simulink model "simulation_model"  (R2022b)
settings: Solver=VariableStepAuto  StartTime=0.0  StopTime=1230000  RelTol=1e-3
model workspace (MAT data in the model file):
  cl1 = 125
  cl2 = 40
  cl3 = 30
  dcmax = [2.05 6.15]
  dcmax2 = [2.04 4]
  iba = 10
undefined symbols (not defined in the file or in its folder): Batt, BatteryCback, BatteryLoadFcn, Continuous, DiscIntNeverNeededParam, gcbh, sps_rtmsupport, spsBatteryModel, Ts
libraries: simulink x7, simulink_extras x2, spsControlledVoltageSourceLib x1, spsCurrentMeasurementLib x1, spsSeriesRLCBranchLib x1, spsControlledCurrentSourceLib x1, spspowerguiLib x1
settings Model: Creator=DSPR_Lab1  LastModifiedBy=DSPR_Lab1

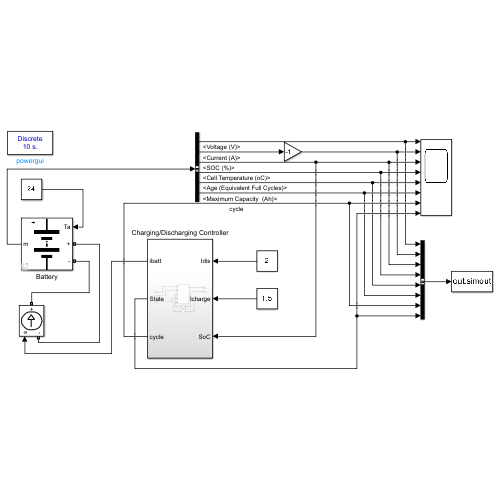
[thumbnail: Simulink's stored preview of the top-level diagram]
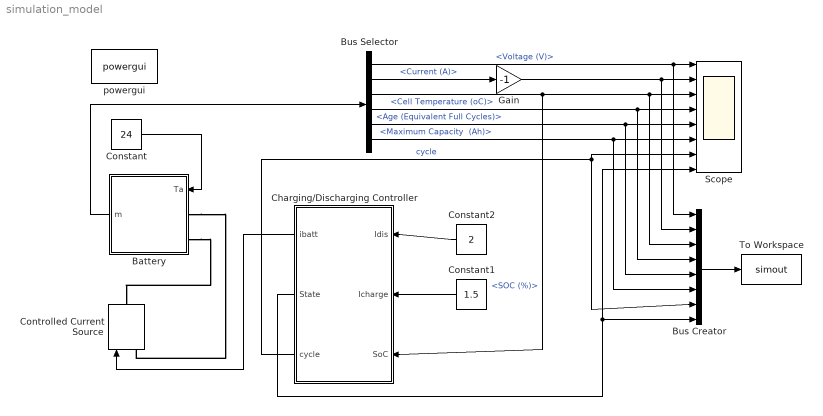
== system simulation_model ==
  Battery : Subsystem  AncestorBlock=sps_lib/Sources/Battery  DialogController=POWERSYS.PowerSysDialog  LoadFcn=sps_rtmsupport('LoadFcn',gcbh); BatteryLoadFcn(gcb)  InitFcn=BatteryCback(gcb,1)  StartFcn=sps_rtmsupport('StartFcn',gcbh);  StopFcn=sps_rtmsupport('StopFcn',gcbh);  mask(Battery){BatType=Lithium-Ion, ShowTempParam=on, ThermalPreset=no, ShowAgeParam=on, NomV=3.3, NomQ=2.05, SOC=0, Batt_Tr=30, PresetModel=off, MaxQ=2.05, MinV=2.75, FullV=4.2, Dis_rate=2, R=.02, Normal_OP=1.9, expZone=[3.38 1.7], current=[.5125 1.025 2.05 4.1 8.2], Units=Ampere-hour, Tci=24, NomT=20, T2=0, MaxQ2=1.85, FullV2=4.1, Normal_OP2=3.3, expZone2=[3.45  1.1], Rca=3, ti=1000, Dp=0, Neq0=iba, Tsim=90, Ta1=20, Qeol=1.49, Reol=0.02*3.2, Char_age=[1.44, 2], Dis_age=[2  6.15], N1=cl1, N2=1600, N3=50, N4=cl2, Ta2=45, N5=cl3}
      mask prompts: BatType "Type:"; ShowTempParam "Simulate temperature effects"; ThermalPreset "Use a preset battery:"; ShowAgeParam "Simulate aging effects"; NomV "Nominal voltage (V)"; NomQ "Rated capacity (Ah)"; SOC "Initial state-of-charge (%)"; Batt_Tr "Battery response time (s)"; PresetModel "Determined from the nominal parameters of the battery"; MaxQ "Maximum capacity (Ah)"; MinV "Cut-off Voltage (V)"; FullV "Fully charged voltage (V)"; Dis_rate "Nominal discharge current (A)"; R "Internal resistance (Ohms)"; Normal_OP "Capacity (Ah) at nominal voltage"; expZone "Exponential zone [Voltage (V), Capacity (Ah)]"; current "Discharge current [i1, i2, i3,...] (A)"; Tci "Initial cell temperature (deg. C)"; NomT "Nominal ambient temperature T1 (deg. C)"; T2 "Second ambient temperature T2 (deg. C)"; MaxQ2 "Maximum capacity (Ah)"; FullV2 "Initial discharge voltage (V)"; Normal_OP2 "Voltage at 90% maximum capacity (V)"; expZone2 "Exponential zone [Voltage (V), Capacity (Ah)]"; Rca "Thermal resistance, cell-to-ambient (deg. C/W)"; ti "Thermal time constant, cell-to-ambient (s)"; Dp "Heat loss difference [charge vs. discharge] (W)"; Neq0 "Initial battery age (Equivalent full cycles)"; Tsim "Aging model sampling time (s)"; Ta1 "Ambient temperature Ta1 (deg. C)"; Qeol "Capacity at EOL (End Of Life) (Ah)"; Reol "Internal resistance at EOL (Ohms)"; Char_age "Charge current (nominal, maximum) [Ic (A), Icmax (A)]"; Dis_age "Discharge current (nominal, maximum) [Id (A), Idmax (A)]"; N1 "Cycle life at 100 % DOD, Ic and Id (Cycles)"; N2 "Cycle life at 25 % DOD, Ic and Id (Cycles)"; N3 "Cycle life at 100 % DOD, Ic and Idmax (Cycles)"; N4 "Cycle life at 100 % DOD, Icmax and Id (Cycles)"; Ta2 "Ambient temperature Ta2 (deg. C)"; N5 "Cycle life at 100 % DOD, Ic and Id (Cycles)"
      mask help: Implements a generic battery model for most popular battery types. Temperature and aging (due to cycling) effects can be specified for Lithium-Ion battery type.
      mask init:
      | block = gcb;
      | BatteryCback(block,3)
      | [Batt BT, WantBlockChoice, Ts] = BatteryParam(NomV,NomQ,MaxQ,MinV,FullV,Dis_rate,R,Normal_OP,expZone,block,0);
      | powericon('SetInternalModels','set',block,WantBlockChoice);
      | BatteryCback(block,1);
      settings: LibrarySourceBlock=sps_lib/Sources/Battery  CopyFcn=sps_rtmsupport('CopyFcn',gcbh);  DeleteFcn=sps_rtmsupport('DeleteFcn',gcbh);  UndoDeleteFcn=sps_rtmsupport('UndoDeleteFcn',gcbh);  ModelCloseFcn=sps_rtmsupport('ModelCloseFcn',gcbh);  PreSaveFcn=sps_rtmsupport('PreSaveFcn',gcbh);  PostSaveFcn=sps_rtmsupport('PostSaveFcn',gcbh);  NameChangeFcn=sps_rtmsupport('NameChangeFcn',gcbh);  PreCopyFcn=sps_rtmsupport('PreCopyFcn',gcbh);  OpenFcn=sps_rtmsupport('OpenFcn',gcbh, [1,2,3,4,9,18]);  CloseFcn=sps_rtmsupport('CloseFcn',gcbh);  PreDeleteFcn=sps_rtmsupport('PreDeleteFcn',gcbh);
      mask Help: helpview(psbhelp)
      mask TypeOptions BatType: Lead-Acid | Lithium-Ion | Nickel-Cadmium | Nickel-Metal-Hydride
      mask Callback BatType: BatteryCback(gcb,1)
      mask Callback ShowTempParam: BatteryCback(gcb,1)
      mask TypeOptions ThermalPreset: no | 3.3V  2.3Ah  (LiFePO4) | 3.6V  2050mAh   (LiCoO2) | 3.6V  2.0Ah | 3.6V  3.6Ah  (LiNiO2) | 3.6V  4.5Ah | 3.6V  48Ah  (LiNiO2) | 3.7V  4.4Ah | 7.4V  5.4Ah  (LiCoO2) | 11.1V  6600mAh  (LiCoO2) | 12.8V  40Ah  (LiFeMgPO4)
      mask Callback ThermalPreset: BatteryCback(gcb,4)
      mask Callback ShowAgeParam: BatteryCback(gcb,1)
      mask Callback PresetModel: BatteryCback(gcb,1)
      mask TypeOptions Units: Ampere-hour | Time
      mask Callback ti: sps_rtmsupport('parametereditingmodes',gcbh, [1,2,3,4,9,18]);
      mask DialogControl ParameterTabVar0 Prompt: Parameters
      mask DialogControl Tempcontainer Prompt: Temperature
      mask DialogControl Agecontainer Prompt: Aging
      mask DialogControl ParameterTabVar01 Prompt: Discharge
      mask DialogControl Container9 Prompt: Display characteristics
      mask DialogControl PlotButton Prompt: Plot
      mask DialogControl PlotButton Callback: BatteryCback(gcb,0)
      mask DialogControl Temperature Prompt: Temperature
      mask DialogControl Container7 Prompt: Discharge parameters at T2
      mask DialogControl Container8 Prompt: Thermal response and Heat loss
      mask DialogControl Aging Prompt: Aging
      mask DialogControl Container16 Prompt: Aging characteristics at ambient temperature Ta1
      mask DialogControl Container13 Prompt: Aging characteristics at ambient temperature Ta2
  Bus Creator : BusCreator  Inputs=8
  Bus Selector : BusSelector  OutputSignals="Voltage (V),Current (A),SOC (%),Cell Temperature (oC),Age (Equivalent Full Cycles),Maximum Capacity  (Ah)"
  Charging/Discharging Controller : Subsystem
  Constant : Constant  Value=24
  Constant1 : Constant  Value=1.5
  Constant2 : Constant  Value=2
  Controlled Current Source : spsControlledCurrentSourceLib/Controlled Current Source  Initialize=on  Source_Type=AC  Amplitude=0  Phase=0  Frequency=0  Measurements=None
  Gain : Gain  Gain=-1
  Scope : Scope  NumInputPorts=8
  To Workspace : ToWorkspace  VariableName=simout  SampleTime=-1
  powergui : spspowerguiLib/powergui  Priority=1  SimulationMode=Discrete  SampleTime=10  frequency=60  Iterations=50  frequencyindice=0  Pbase=100e6  ErrMax=1e-4  UnitsV=kV  UnitsW=MW  buscounter=0  FunctionMessages=off  echomessages=off  EnableUseOfTLC=off  CurrentSourceSwitches=on  DisableSnubberDevices=off  DisableRonSwitches=off  DisableVfSwitches=off  DisplayEquations=off  AutomaticDiscreteSolvers=off  SolverType=Tustin/Backward Euler (TBE)  Interpol=off  ExternalGateDelay=off  methode=off  Ts=100  x0status=blocks  SPID=on  SwTol=0  HookPort=off  NonlinearTolerance=1e-4  nMaxIteration=100  ContinueOnMaxIteration=off  RestoreLinks=warning  ResistiveCurrentMeasurement=off  Frange=[0:2:500]  Ylog=off  Xlog=on  ShowGrid=off  save=off  variable=ZData  structure=0  ZoomFFT=off  StartTime=0.0  cycles=1  DisplayStyle=1  fundamental=60  FreqAxis=off  MaxFrequency=1000  frequencyindicesteady=1  RmsSteady=1  display=off
  wires:
  Charging/Discharging Controller/3(cycle) -> Bus Creator/7, Scope/7  "cycle"
  Bus Selector/2 -> Gain/1  "<Current (A)>"
  Charging/Discharging Controller/2(State) -> Scope/8, Bus Creator/8
  Constant1/1 -> Charging/Discharging Controller/2(Icharge)
  Constant/1 -> Battery/1(Ta)
  Charging/Discharging Controller/1(ibatt) -> Controlled Current Source/1
  Constant2/1 -> Charging/Discharging Controller/1(Idis)
  Bus Creator/1 -> To Workspace/1
  Battery/1(m) -> Bus Selector/1
  Bus Selector/1 -> Bus Creator/1, Scope/1  "<Voltage (V)>"
  Gain/1 -> Bus Creator/2, Scope/2
  Bus Selector/3 -> Charging/Discharging Controller/3(SoC), Bus Creator/3, Scope/3  "<SOC (%)>"
  Bus Selector/4 -> Bus Creator/4, Scope/4  "<Cell Temperature (oC)>"
  Bus Selector/5 -> Bus Creator/5, Scope/5  "<Age (Equivalent Full Cycles)>"
  Bus Selector/6 -> Bus Creator/6, Scope/6  "<Maximum Capacity  (Ah)>"
  connections:
  Battery/LConn2 -- Controlled Current Source/RConn1
  Battery/LConn1 -- Controlled Current Source/LConn1

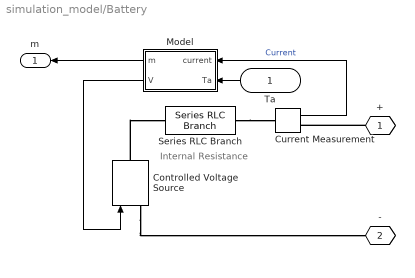
== system simulation_model/Battery ==
  note: Internal Resistance
  Ta : Inport
  Controlled Voltage Source : spsControlledVoltageSourceLib/Controlled Voltage Source  Initialize=on  Source_Type=AC  Amplitude=0  Phase=0  Frequency=0  Measurements=None
  Current Measurement : spsCurrentMeasurementLib/Current Measurement  PhasorSimulation=off  OutputType=Complex  PSBequivalent=0
  Model : Subsystem  AncestorBlock=spsBatteryModel/Continuous
      settings: LibrarySourceBlock=spsBatteryModel/Continuous
  Series RLC Branch : spsSeriesRLCBranchLib/Series RLC Branch  LConnTagsString=__new0  RConnTagsString=__new0  BranchType=R  Resistance=Batt.R  Inductance=1e-3  SetiL0=off  InitialCurrent=0  Capacitance=1e-6  Setx0=off  InitialVoltage=0  Measurements=None
  + : PMIOPort  Tag=PMCPort  Side=Left
  - : PMIOPort  Tag=PMCPort  Port=2  Side=Left
  m : Outport  VectorParamsAs1DForOutWhenUnconnected=off
  wires:
  Model/2(V) -> Controlled Voltage Source/1
  Model/1(m) -> m/1
  Current Measurement/1 -> Model/1(current)  "Current"
  Ta/1 -> Model/2(Ta)
  connections:
  +/RConn1 -- Current Measurement/RConn1
  Controlled Voltage Source/LConn1 -- -/RConn1
  Controlled Voltage Source/RConn1 -- Series RLC Branch/LConn1
  Series RLC Branch/RConn1 -- Current Measurement/LConn1

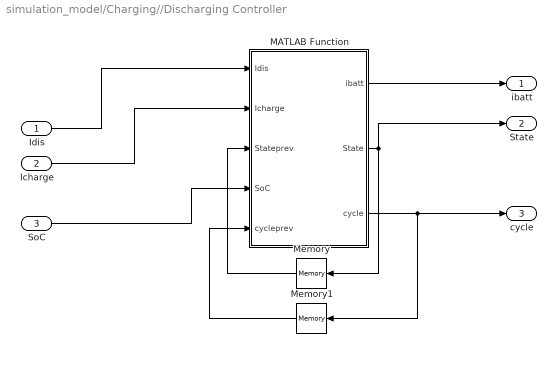
== system simulation_model/Charging//Discharging Controller ==
  Idis : Inport
  Icharge : Inport  Port=2
  SoC : Inport  Port=3
  MATLAB Function : MATLAB Function  TreatAsAtomicUnit=on
  Memory : Memory
  Memory1 : Memory
  ibatt : Outport
  State : Outport  Port=2
  cycle : Outport  Port=3
  wires:
  Idis/1 -> MATLAB Function/1(Idis)
  Icharge/1 -> MATLAB Function/2(Icharge)
  Memory/1 -> MATLAB Function/3(Stateprev)
  MATLAB Function/2(State) -> Memory/1, State/1
  MATLAB Function/1(ibatt) -> ibatt/1
  SoC/1 -> MATLAB Function/4(SoC)
  MATLAB Function/3(cycle) -> cycle/1, Memory1/1
  Memory1/1 -> MATLAB Function/5(cycleprev)

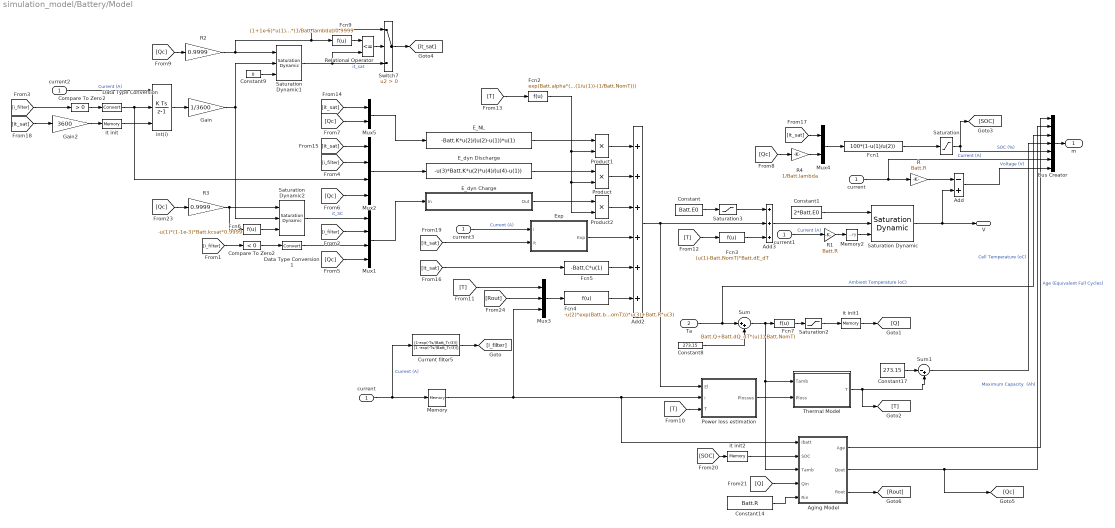
== system simulation_model/Battery/Model ==
  current : Inport
  Ta : Inport  Port=2
  Add : Sum  Inputs=-+
  Add2 : Sum  Inputs=++++++
  Add3 : Sum  Inputs=+++
  Aging Model : Subsystem  AncestorBlock=spsBatteryModel/Aging Model
      settings: LibrarySourceBlock=spsBatteryModel/Aging Model
  Bus Creator : BusCreator  Inputs=7
  Compare To Zero : simulink/Logic and Bit Operations/Compare To Zero  relop=>  OutDataTypeStr=uint8
  Compare To Zero2 : simulink/Logic and Bit Operations/Compare To Zero  relop=<  OutDataTypeStr=uint8
  Constant : Constant  Value=Batt.E0
  Constant1 : Constant  Value=2*Batt.E0
  Constant14 : Constant  Value=Batt.R
  Constant17 : Constant  Value=273.15
  Constant8 : Constant  Value=273.15
  Constant9 : Constant  Value=0
  Current filter5 : DiscreteTransferFcn  Numerator=[1-exp(-Ts/(Batt_Tr/3))]  Denominator=[1 -exp(-Ts/(Batt_Tr/3))]  SampleTime=Ts
  Data Type Conversion1 : DataTypeConversion  SaturateOnIntegerOverflow=off  RndMeth=Floor
  Data Type Conversion2 : DataTypeConversion  SaturateOnIntegerOverflow=off  RndMeth=Floor
  E_NL : Fcn  Expr=-Batt.K*u(2)/(u(2)-u(1))*u(1)
  E_dyn Charge : Subsystem
  E_dyn Discharge : Fcn  Expr=-u(3)*Batt.K*u(2)*u(4)/(u(4)-u(1))
  Exp : Subsystem
  Fcn1 : Fcn  Expr=100*(1-u(1)/u(2))
  Fcn2 : Fcn  Expr=exp(Batt.alpha*((1/u(1))-(1/Batt.NomT)))
  Fcn3 : Fcn  Expr=(u(1)-Batt.NomT)*Batt.dE_dT
  Fcn4 : Fcn  Expr=-u(2)*exp(Batt.beta*((1/u(1))-(1/Batt.NomT)))*u(3)+Batt.R*u(3)
  Fcn5 : Fcn  Expr=-Batt.C*u(1)
  Fcn6 : Fcn  Expr=-u(1)*(1-1e-3)*Batt.kcsat*0.9999
  Fcn7 : Fcn  Expr=Batt.Q+Batt.dQ_dT*(u(1)-Batt.NomT)
  Fcn9 : Fcn  Expr=(1+1e-6)*u(1)*(1/Batt.lambda)/0.9999
  Gain : Gain  Gain=1/3600
  Gain2 : Gain  Gain=3600
  Memory : Memory
  Memory2 : Memory  InheritSampleTime=on
  Mux1 : Mux
  Mux2 : Mux
  Mux3 : Mux  Inputs=3
  Mux4 : Mux  Inputs=2
  Mux5 : Mux  Inputs=2
  Power loss estimation : Subsystem
  Product : Product
  Product1 : Product
  Product2 : Product
  R : Gain  Gain=Batt.R
  R1 : Gain  Gain=Batt.R
  R2 : Gain  Gain=0.9999
  R3 : Gain  Gain=0.9999
  R4 : Gain  Gain=1/Batt.lambda
  Relational Operator : RelationalOperator  Operator=<=  RndMeth=Simplest  InputSameDT=off
  Saturation : Saturate  UpperLimit=100  LowerLimit=0
  Saturation Dynamic : simulink/Discontinuities/Saturation Dynamic  OutMin=[]  OutMax=[]  OutDataTypeStr=Inherit: Same as second input  OutDataType=sfix(16)  OutScaling=2^-10  DoSatur=off
  Saturation Dynamic1 : simulink/Discontinuities/Saturation Dynamic  OutMin=[]  OutMax=[]  OutDataTypeStr=Inherit: Same as second input  OutDataType=sfix(16)  OutScaling=2^-10  DoSatur=off
  Saturation Dynamic2 : simulink/Discontinuities/Saturation Dynamic  OutMin=[]  OutMax=[]  OutDataTypeStr=Inherit: Same as second input  OutDataType=sfix(16)  OutScaling=2^-10  DoSatur=off
  Saturation2 : Saturate  UpperLimit=max(NomQ,MaxQ)  LowerLimit=0
  Saturation3 : Saturate  UpperLimit=Batt.Va-Batt.dE_dT*(Batt.Tci-Batt.NomT)-Batt.A  LowerLimit=-inf
  Sum : Sum  Inputs=|++
  Sum1 : Sum  Inputs=|-+
  Switch7 : Switch  Criteria=u2 > Threshold  SaturateOnIntegerOverflow=off  InputSameDT=off
  Thermal Model : Subsystem  VariantControl=Discrete
  "current " : InportShadow
  current1 : InportShadow
  current2 : InportShadow
  current3 : InportShadow
  int(i) : DiscreteIntegrator  ExternalReset=rising  InitialConditionSource=external  SampleTime=Ts  LimitOutput=on  UpperSaturationLimit=Batt.Qmax*3600  ICPrevOutput=DiscIntNeverNeededParam  ICPrevScaledInput=DiscIntNeverNeededParam
  it init : Memory  InitialCondition=(1-SOC/100)*Batt.Q*(1/Batt.lambda)*3600
  it init1 : Memory  InitialCondition=MaxQ
  it init2 : Memory  InitialCondition=SOC
  m : Outport  VectorParamsAs1DForOutWhenUnconnected=off
  V : Outport  Port=2  VectorParamsAs1DForOutWhenUnconnected=off
  wires:
  current/1 -> Bus Creator/6, R/1  "Current (A)"
  int(i)/1 -> Gain/1
  Fcn1/1 -> Saturation/1
  Add/1 -> Bus Creator/7  "Voltage (V)"
  R/1 -> Add/1
  Bus Creator/1 -> m/1
  Mux2/1 -> E_dyn Discharge/1
  Constant/1 -> Saturation3/1
  Mux1/1 -> E_dyn Charge/1(In)
  it init/1 -> int(i)/3
  Compare To Zero/1 -> Data Type Conversion2/1
  Compare To Zero2/1 -> Data Type Conversion1/1
  Data Type Conversion2/1 -> Mux2/3, int(i)/2
  Gain2/1 -> it init/1
  Exp/1(Exp) -> Add2/4
  Data Type Conversion1/1 -> Mux1/3
  Saturation Dynamic2/1 -> Mux1/1  "it_SC"
  Constant1/1 -> Saturation Dynamic/1
  Add3/1 -> Saturation Dynamic/2
  E_dyn Discharge/1 -> Product/1
  Product/1 -> Add2/2
  E_NL/1 -> Product1/1
  Product1/1 -> Add2/1
  Memory/1 -> Mux3/3, Aging Model/1(Ibatt), Power loss estimation/2(i)
  Power loss estimation/1(Plosses) -> Thermal Model/2(Ploss)
  Fcn2/1 -> Product2/2, Product/2, Product1/2
  Fcn4/1 -> Add2/6
  Mux3/1 -> Fcn4/1
  E_dyn Charge/1(Out) -> Product2/1
  Product2/1 -> Add2/3
  Fcn5/1 -> Add2/5
  Ta/1 -> Sum/1, Bus Creator/3  "Ambient Temperature (oC)"
  Constant8/1 -> Sum/2
  Mux4/1 -> Fcn1/1
  Mux5/1 -> E_NL/1
  Fcn3/1 -> Add3/3
  Fcn6/1 -> Saturation Dynamic2/3
  Sum/1 -> Aging Model/3(Tamb), Thermal Model/1(Tamb), Fcn7/1
  Fcn7/1 -> Saturation2/1
  Saturation3/1 -> Add3/1
  Saturation2/1 -> it init1/1
  current2/1 -> int(i)/1  "Current (A)"
  current3/1 -> Exp/1(i)  "Current (A)"
  "current "/1 -> Current filter5/1, Memory/1  "Current (A)"
  Current filter5/1 -> [i_filter]
  [i_filter] -> Compare To Zero2/1
  [i_filter] -> Mux1/2
  [i_filter] -> Compare To Zero/1
  [i_filter] -> Mux2/2
  it init1/1 -> [Q]
  [Qc] -> Mux1/4
  [Qc] -> Mux2/4
  [Qc] -> R4/1
  [Qc] -> R2/1
  [T] -> Mux3/1
  [T] -> Fcn3/1
  [T] -> Fcn2/1
  [it_sat] -> Mux5/1
  [it_sat] -> Mux2/1
  [it_sat] -> Fcn5/1
  [it_sat] -> Mux4/1
  [it_sat] -> Gain2/1
  [it_sat] -> Exp/2(it)
  [Qc] -> R3/1
  R3/1 -> Fcn6/1, Saturation Dynamic2/1
  Add2/1 -> Power loss estimation/1(El), Add3/2
  [T] -> Power loss estimation/3(T)
  R4/1 -> Mux4/2
  Saturation/1 -> Bus Creator/5, [SOC]  "SOC (%)"
  Saturation Dynamic/1 -> V/1, Add/2
  [Qc] -> Mux5/2
  [SOC] -> it init2/1
  [Q] -> Aging Model/4(Qin)
  Aging Model/2(Qout) -> Bus Creator/2, [Qc]  "Maximum Capacity  (Ah)"
  Constant14/1 -> Aging Model/5(Rin)
  Aging Model/3(Rout) -> [Rout]
  [Rout] -> Mux3/2
  Aging Model/1(Age) -> Bus Creator/1  "Age (Equivalent Full Cycles)"
  it init2/1 -> Aging Model/2(SOC)
  Gain/1 -> Saturation Dynamic1/2, Saturation Dynamic2/2
  Constant9/1 -> Saturation Dynamic1/3
  current1/1 -> R1/1  "Current (A)"
  Memory2/1 -> Saturation Dynamic/3
  R1/1 -> Memory2/1
  Saturation Dynamic1/1 -> Relational Operator/2, Switch7/3  "it_sat"
  R2/1 -> Switch7/1, Fcn9/1, Saturation Dynamic1/1
  Switch7/1 -> [it_sat]
  Fcn9/1 -> Relational Operator/1
  Relational Operator/1 -> Switch7/2
  Constant17/1 -> Sum1/1
  Thermal Model/1(T) -> Sum1/2, [T]
  Sum1/1 -> Bus Creator/4  "Cell Temperature (oC)"

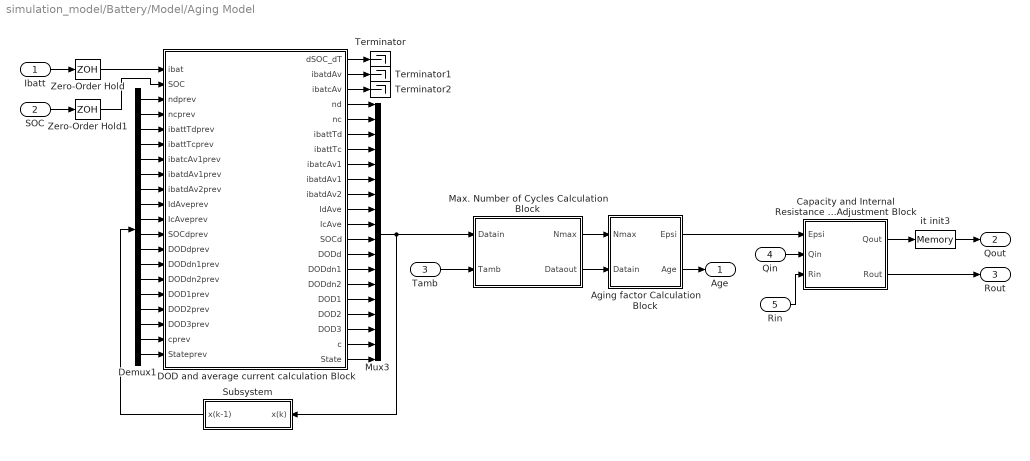
== system simulation_model/Battery/Model/Aging Model ==
  Ibatt : Inport
  SOC : Inport  Port=2
  Tamb : Inport  Port=3
  Qin : Inport  Port=4
  Rin : Inport  Port=5
  Aging factor Calculation Block : Subsystem
  Capacity and Internal Resistance Adjustment Block : Subsystem
  DOD and average current calculation Block : MATLAB Function  TreatAsAtomicUnit=on
  Demux1 : Demux  Outputs=18
      settings: DisplayOption=none
  Max. Number of Cycles Calculation Block : Subsystem
  Mux3 : Mux  Inputs=18
  Subsystem : Subsystem
  Terminator : Terminator
  Terminator1 : Terminator
  Terminator2 : Terminator
  Zero-Order Hold : ZeroOrderHold  SampleTime=Batt.Tsim
  Zero-Order Hold1 : ZeroOrderHold  SampleTime=Batt.Tsim
  it init3 : Memory  InitialCondition=MaxQ
  Age : Outport  VectorParamsAs1DForOutWhenUnconnected=off
  Qout : Outport  Port=2  VectorParamsAs1DForOutWhenUnconnected=off
  Rout : Outport  Port=3  VectorParamsAs1DForOutWhenUnconnected=off
  wires:
  it init3/1 -> Qout/1
  Zero-Order Hold1/1 -> DOD and average current calculation Block/2(SOC)
  Zero-Order Hold/1 -> DOD and average current calculation Block/1(ibat)
  Aging factor Calculation Block/2(Age) -> Age/1
  SOC/1 -> Zero-Order Hold1/1
  Ibatt/1 -> Zero-Order Hold/1
  Max. Number of Cycles Calculation Block/2(Dataout) -> Aging factor Calculation Block/2(Datain)
  Max. Number of Cycles Calculation Block/1(Nmax) -> Aging factor Calculation Block/1(Nmax)
  Demux1/5 -> DOD and average current calculation Block/7(ibatcAv1prev)
  DOD and average current calculation Block/2(ibatdAv) -> Terminator1/1
  DOD and average current calculation Block/3(ibatcAv) -> Terminator2/1
  DOD and average current calculation Block/1(dSOC_dT) -> Terminator/1
  Demux1/2 -> DOD and average current calculation Block/4(ncprev)
  Subsystem/1(x(k-1)) -> Demux1/1
  Demux1/1 -> DOD and average current calculation Block/3(ndprev)
  DOD and average current calculation Block/18(DOD2) -> Mux3/15
  DOD and average current calculation Block/12(IcAve) -> Mux3/9
  DOD and average current calculation Block/17(DOD1) -> Mux3/14
  Demux1/8 -> DOD and average current calculation Block/10(IdAveprev)
  Demux1/14 -> DOD and average current calculation Block/16(DOD1prev)
  DOD and average current calculation Block/8(ibatcAv1) -> Mux3/5
  Demux1/4 -> DOD and average current calculation Block/6(ibattTcprev)
  DOD and average current calculation Block/7(ibattTc) -> Mux3/4
  DOD and average current calculation Block/11(IdAve) -> Mux3/8
  DOD and average current calculation Block/19(DOD3) -> Mux3/16
  DOD and average current calculation Block/10(ibatdAv2) -> Mux3/7
  DOD and average current calculation Block/14(DODd) -> Mux3/11
  Demux1/7 -> DOD and average current calculation Block/9(ibatdAv2prev)
  Demux1/15 -> DOD and average current calculation Block/17(DOD2prev)
  DOD and average current calculation Block/6(ibattTd) -> Mux3/3
  Demux1/11 -> DOD and average current calculation Block/13(DODdprev)
  DOD and average current calculation Block/20(c) -> Mux3/17
  Demux1/18 -> DOD and average current calculation Block/20(Stateprev)
  DOD and average current calculation Block/13(SOCd) -> Mux3/10
  DOD and average current calculation Block/21(State) -> Mux3/18
  DOD and average current calculation Block/15(DODdn1) -> Mux3/12
  DOD and average current calculation Block/5(nc) -> Mux3/2
  Demux1/17 -> DOD and average current calculation Block/19(cprev)
  Demux1/16 -> DOD and average current calculation Block/18(DOD3prev)
  Demux1/9 -> DOD and average current calculation Block/11(IcAveprev)
  Demux1/12 -> DOD and average current calculation Block/14(DODdn1prev)
  Demux1/6 -> DOD and average current calculation Block/8(ibatdAv1prev)
  DOD and average current calculation Block/16(DODdn2) -> Mux3/13
  DOD and average current calculation Block/4(nd) -> Mux3/1
  Demux1/13 -> DOD and average current calculation Block/15(DODdn2prev)
  Demux1/3 -> DOD and average current calculation Block/5(ibattTdprev)
  Demux1/10 -> DOD and average current calculation Block/12(SOCdprev)
  DOD and average current calculation Block/9(ibatdAv1) -> Mux3/6
  Tamb/1 -> Max. Number of Cycles Calculation Block/2(Tamb)
  Capacity and Internal Resistance Adjustment Block/1(Qout) -> it init3/1
  Qin/1 -> Capacity and Internal Resistance Adjustment Block/2(Qin)
  Rin/1 -> Capacity and Internal Resistance Adjustment Block/3(Rin)
  Capacity and Internal Resistance Adjustment Block/2(Rout) -> Rout/1
  Aging factor Calculation Block/1(Epsi) -> Capacity and Internal Resistance Adjustment Block/1(Epsi)
  Mux3/1 -> Max. Number of Cycles Calculation Block/1(Datain), Subsystem/1(x(k))

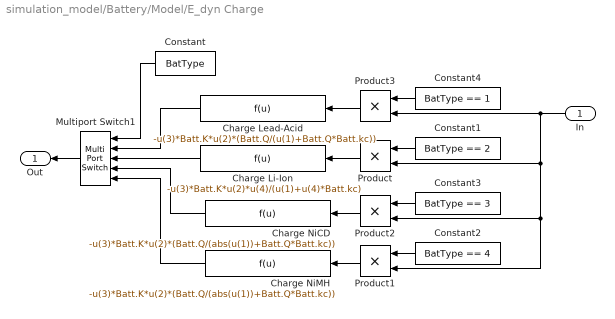
== system simulation_model/Battery/Model/E_dyn Charge ==
  In : Inport
  Charge Lead-Acid : Fcn  Expr=-u(3)*Batt.K*u(2)*(Batt.Q/(u(1)+Batt.Q*Batt.kc))
  Charge Li-Ion : Fcn  Expr=-u(3)*Batt.K*u(2)*u(4)/(u(1)+u(4)*Batt.kc)
  Charge NiCD : Fcn  Expr=-u(3)*Batt.K*u(2)*(Batt.Q/(abs(u(1))+Batt.Q*Batt.kc))
  Charge NiMH : Fcn  Expr=-u(3)*Batt.K*u(2)*(Batt.Q/(abs(u(1))+Batt.Q*Batt.kc))
  Constant : Constant  Value=BatType
  Constant1 : Constant  Value=BatType == 2  OutDataTypeStr=double
  Constant2 : Constant  Value=BatType == 4  OutDataTypeStr=double
  Constant3 : Constant  Value=BatType == 3  OutDataTypeStr=double
  Constant4 : Constant  Value=BatType == 1  OutDataTypeStr=double
  Multiport Switch1 : MultiPortSwitch  Inputs=4  SaturateOnIntegerOverflow=off  InputSameDT=off
  Product{,1..3} (4 alike) : Product  RndMeth=Zero
  Out : Outport  VectorParamsAs1DForOutWhenUnconnected=off
  wires:
  Multiport Switch1/1 -> Out/1
  Charge Li-Ion/1 -> Multiport Switch1/3
  Charge NiMH/1 -> Multiport Switch1/5
  Charge NiCD/1 -> Multiport Switch1/4
  Charge Lead-Acid/1 -> Multiport Switch1/2
  Constant/1 -> Multiport Switch1/1
  In/1 -> Product3/2, Product/2, Product1/2, Product2/2
  Product/1 -> Charge Li-Ion/1
  Constant1/1 -> Product/1
  Product1/1 -> Charge NiMH/1
  Constant2/1 -> Product1/1
  Product2/1 -> Charge NiCD/1
  Constant3/1 -> Product2/1
  Product3/1 -> Charge Lead-Acid/1
  Constant4/1 -> Product3/1

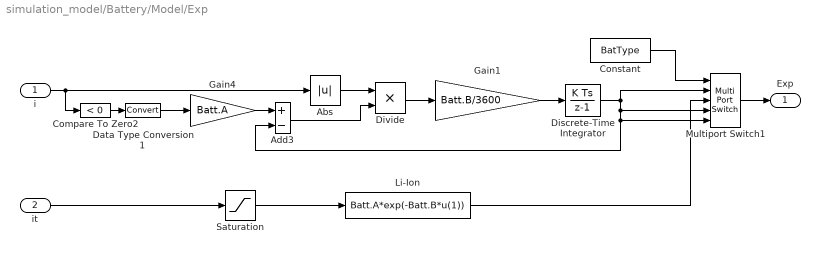
== system simulation_model/Battery/Model/Exp ==
  i : Inport
  it : Inport  Port=2
  Abs : Abs  SaturateOnIntegerOverflow=off
  Add3 : Sum  Inputs=+-
  Compare To Zero2 : simulink/Logic and Bit Operations/Compare To Zero  relop=<  OutDataTypeStr=uint8
  Constant : Constant  Value=BatType
  Data Type Conversion1 : DataTypeConversion  SaturateOnIntegerOverflow=off  RndMeth=Floor
  Discrete-Time Integrator : DiscreteIntegrator  InitialCondition=Batt.A*exp(-Batt.B*(1-SOC/100)*Batt.Q)  SampleTime=Ts  ICPrevOutput=DiscIntNeverNeededParam  ICPrevScaledInput=DiscIntNeverNeededParam
  Divide : Product  Inputs=**
  Gain1 : Gain  Gain=Batt.B/3600
  Gain4 : Gain  Gain=Batt.A
  Li-Ion : Fcn  Expr=Batt.A*exp(-Batt.B*u(1))
  Multiport Switch1 : MultiPortSwitch  Inputs=4  SaturateOnIntegerOverflow=off  InputSameDT=off
  Saturation : Saturate  UpperLimit=Batt.Qmax*(1/Batt.lambda)  LowerLimit=-inf
  Exp : Outport  VectorParamsAs1DForOutWhenUnconnected=off
  wires:
  Discrete-Time Integrator/1 -> Multiport Switch1/2, Multiport Switch1/4, Add3/2, Multiport Switch1/5
  Gain4/1 -> Add3/1
  Divide/1 -> Gain1/1
  Abs/1 -> Divide/1
  Add3/1 -> Divide/2
  Gain1/1 -> Discrete-Time Integrator/1
  i/1 -> Abs/1, Compare To Zero2/1
  Constant/1 -> Multiport Switch1/1
  it/1 -> Saturation/1
  Li-Ion/1 -> Multiport Switch1/3
  Multiport Switch1/1 -> Exp/1
  Compare To Zero2/1 -> Data Type Conversion1/1
  Data Type Conversion1/1 -> Gain4/1
  Saturation/1 -> Li-Ion/1

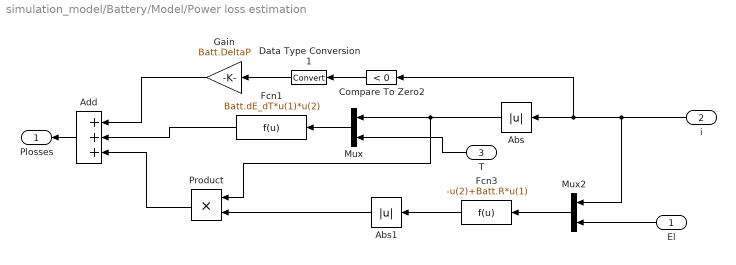
== system simulation_model/Battery/Model/Power loss estimation ==
  El : Inport
  i : Inport  Port=2
  T : Inport  Port=3
  Abs : Abs  SaturateOnIntegerOverflow=off
  Abs1 : Abs  SaturateOnIntegerOverflow=off
  Add : Sum  Inputs=+++
  Compare To Zero2 : simulink/Logic and Bit Operations/Compare To Zero  relop=<  OutDataTypeStr=uint8
  Data Type Conversion1 : DataTypeConversion  SaturateOnIntegerOverflow=off  RndMeth=Floor
  Fcn1 : Fcn  Expr=Batt.dE_dT*u(1)*u(2)
  Fcn3 : Fcn  Expr=-u(2)+Batt.R*u(1)
  Gain : Gain  Gain=Batt.DeltaP
  Mux : Mux  Inputs=2
  Mux2 : Mux  Inputs=2
  Product : Product
  Plosses : Outport  VectorParamsAs1DForOutWhenUnconnected=off
  wires:
  i/1 -> Compare To Zero2/1, Abs/1, Mux2/1
  T/1 -> Mux/2
  Add/1 -> Plosses/1
  Mux/1 -> Fcn1/1
  Abs/1 -> Mux/1, Product/1
  Abs1/1 -> Product/2
  El/1 -> Mux2/2
  Fcn3/1 -> Abs1/1
  Mux2/1 -> Fcn3/1
  Product/1 -> Add/3
  Fcn1/1 -> Add/2
  Compare To Zero2/1 -> Data Type Conversion1/1
  Data Type Conversion1/1 -> Gain/1
  Gain/1 -> Add/1

== system simulation_model/Battery/Model/Thermal Model ==
  Tamb : Inport
  Ploss : Inport  Port=2
  Discrete Transfer Fcn (with initial outputs) : simulink_extras/Additional Discrete/Discrete Transfer Fcn (with initial outputs)  N=[1-exp(-Ts/(Batt.tc))]  D=[1 -exp(-Ts/(Batt.tc))]  U0=0  Y0=Batt.Tci  TS=Ts
  Discrete Transfer Fcn (with initial outputs)1 : simulink_extras/Additional Discrete/Discrete Transfer Fcn (with initial outputs)  N=[1-exp(-Ts/1e-6)]  D=[1 -exp(-Ts/1e-6)]  U0=0  Y0=0  TS=Ts
  Gain : Gain  Gain=Batt.Rth
  Sum : Sum  Inputs=|++
  T : Outport  VectorParamsAs1DForOutWhenUnconnected=off
  wires:
  Sum/1 -> Discrete Transfer Fcn (with initial outputs)/1
  Gain/1 -> Sum/2
  Ploss/1 -> Discrete Transfer Fcn (with initial outputs)1/1
  Discrete Transfer Fcn (with initial outputs)/1 -> T/1  "Cell Temperature (K)"
  Discrete Transfer Fcn (with initial outputs)1/1 -> Gain/1
  Tamb/1 -> Sum/1

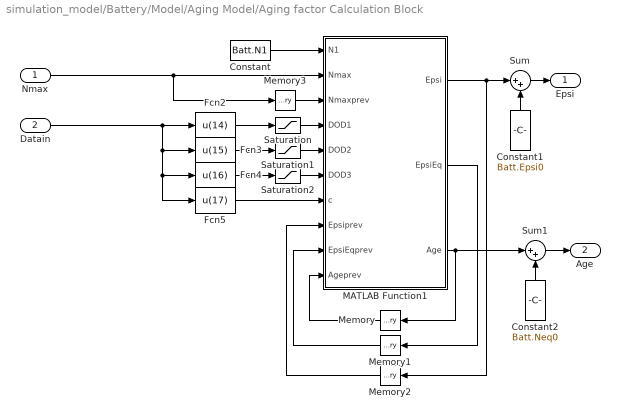
== system simulation_model/Battery/Model/Aging Model/Aging factor Calculation Block ==
  Nmax : Inport
  Datain : Inport  Port=2
  Constant : Constant  Value=Batt.N1
  Constant1 : Constant  Value=Batt.Epsi0
  Constant2 : Constant  Value=Batt.Neq0
  Fcn2 : Fcn  Expr=u(14)
  Fcn3 : Fcn  Expr=u(15)
  Fcn4 : Fcn  Expr=u(16)
  Fcn5 : Fcn  Expr=u(17)
  MATLAB Function1 : MATLAB Function  TreatAsAtomicUnit=on
  Memory{,1..3} (4 alike) : Memory  InheritSampleTime=on
  Saturation : Saturate  UpperLimit=inf  LowerLimit=0.01
  Saturation1 : Saturate  UpperLimit=inf  LowerLimit=0.01
  Saturation2 : Saturate  UpperLimit=inf  LowerLimit=0.01
  Sum : Sum  Inputs=|++
  Sum1 : Sum  Inputs=|++
  Epsi : Outport  VectorParamsAs1DForOutWhenUnconnected=off
  Age : Outport  Port=2  VectorParamsAs1DForOutWhenUnconnected=off
  wires:
  MATLAB Function1/3(Age) -> Memory/1, Sum1/1
  Sum1/1 -> Age/1
  Constant2/1 -> Sum1/2
  Constant1/1 -> Sum/2
  Sum/1 -> Epsi/1
  Memory/1 -> MATLAB Function1/10(Ageprev)
  Fcn5/1 -> MATLAB Function1/7(c)
  Constant/1 -> MATLAB Function1/1(N1)
  Memory1/1 -> MATLAB Function1/9(EpsiEqprev)
  MATLAB Function1/2(EpsiEq) -> Memory1/1
  Saturation/1 -> MATLAB Function1/4(DOD1)
  Memory2/1 -> MATLAB Function1/8(Epsiprev)
  Datain/1 -> Fcn2/1, Fcn4/1, Fcn5/1, Fcn3/1
  Fcn3/1 -> Saturation1/1
  Fcn4/1 -> Saturation2/1
  Saturation1/1 -> MATLAB Function1/5(DOD2)
  Fcn2/1 -> Saturation/1
  Saturation2/1 -> MATLAB Function1/6(DOD3)
  Nmax/1 -> MATLAB Function1/2(Nmax), Memory3/1
  MATLAB Function1/1(Epsi) -> Sum/1, Memory2/1
  Memory3/1 -> MATLAB Function1/3(Nmaxprev)

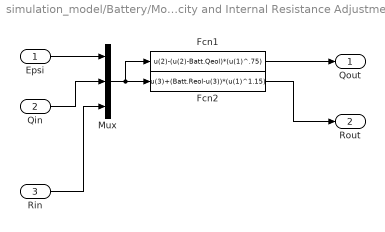
== system simulation_model/Battery/Model/Aging Model/Capacity and Internal Resistance Adjustment Block ==
  Epsi : Inport
  Qin : Inport  Port=2
  Rin : Inport  Port=3
  Fcn1 : Fcn  Expr=u(2)-(u(2)-Batt.Qeol)*(u(1)^.75)
  Fcn2 : Fcn  Expr=u(3)+(Batt.Reol-u(3))*(u(1)^1.15)
  Mux : Mux  Inputs=3
  Qout : Outport  VectorParamsAs1DForOutWhenUnconnected=off
  Rout : Outport  Port=2  VectorParamsAs1DForOutWhenUnconnected=off
  wires:
  Qin/1 -> Mux/2
  Rin/1 -> Mux/3
  Epsi/1 -> Mux/1
  Fcn2/1 -> Rout/1
  Mux/1 -> Fcn2/1, Fcn1/1
  Fcn1/1 -> Qout/1

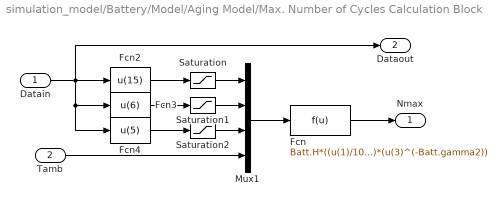
== system simulation_model/Battery/Model/Aging Model/Max. Number of Cycles Calculation Block ==
  Datain : Inport
  Tamb : Inport  Port=2
  Fcn : Fcn  Expr=Batt.H*((u(1)/100)^(-Batt.zeta))*exp(-Batt.phi*((1/Batt.Tref)-(1/u(4))))*(u(2)^(-Batt.gamma1))*(u(3)^(-Batt.gamma2))
  Fcn2 : Fcn  Expr=u(15)
  Fcn3 : Fcn  Expr=u(6)
  Fcn4 : Fcn  Expr=u(5)
  Mux1 : Mux
  Saturation : Saturate  UpperLimit=inf  LowerLimit=0.01
  Saturation1 : Saturate  UpperLimit=inf  LowerLimit=0.01
  Saturation2 : Saturate  UpperLimit=inf  LowerLimit=0.01
  Nmax : Outport  VectorParamsAs1DForOutWhenUnconnected=off
  Dataout : Outport  Port=2  VectorParamsAs1DForOutWhenUnconnected=off
  wires:
  Datain/1 -> Fcn2/1, Fcn3/1, Fcn4/1, Dataout/1
  Mux1/1 -> Fcn/1
  Tamb/1 -> Mux1/4
  Fcn4/1 -> Saturation2/1
  Fcn3/1 -> Saturation1/1
  Saturation/1 -> Mux1/1
  Fcn2/1 -> Saturation/1
  Saturation2/1 -> Mux1/3
  Saturation1/1 -> Mux1/2
  Fcn/1 -> Nmax/1

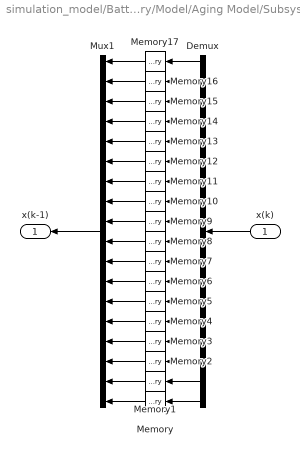
== system simulation_model/Battery/Model/Aging Model/Subsystem ==
  x(k) : Inport
  Demux : Demux  Outputs=18
      settings: DisplayOption=none
  Memory : Memory  InitialCondition=1  InheritSampleTime=on
  Memory{1..7,9..17} (16 alike) : Memory  InheritSampleTime=on
  Memory8 : Memory  InitialCondition=SOC  InheritSampleTime=on
  Mux1 : Mux  Inputs=18
  x(k-1) : Outport  VectorParamsAs1DForOutWhenUnconnected=off
  wires:
  Memory/1 -> Mux1/18
  Memory1/1 -> Mux1/17
  Memory2/1 -> Mux1/16
  Memory3/1 -> Mux1/15
  Memory4/1 -> Mux1/14
  Memory5/1 -> Mux1/13
  Memory6/1 -> Mux1/12
  Memory7/1 -> Mux1/11
  Memory8/1 -> Mux1/10
  Memory9/1 -> Mux1/9
  Memory10/1 -> Mux1/8
  Memory11/1 -> Mux1/7
  Memory12/1 -> Mux1/6
  Memory13/1 -> Mux1/5
  Memory14/1 -> Mux1/4
  Memory16/1 -> Mux1/2
  Memory15/1 -> Mux1/3
  Memory17/1 -> Mux1/1
  Demux/1 -> Memory17/1
  Demux/2 -> Memory16/1
  Demux/3 -> Memory15/1
  Demux/4 -> Memory14/1
  Demux/5 -> Memory13/1
  Demux/6 -> Memory12/1
  Demux/7 -> Memory11/1
  Demux/8 -> Memory10/1
  Demux/9 -> Memory9/1
  Demux/10 -> Memory8/1
  Demux/11 -> Memory7/1
  Demux/12 -> Memory6/1
  Demux/13 -> Memory5/1
  Demux/14 -> Memory4/1
  Demux/15 -> Memory3/1
  Demux/16 -> Memory2/1
  Demux/17 -> Memory1/1
  Demux/18 -> Memory/1
  x(k)/1 -> Demux/1
  Mux1/1 -> x(k-1)/1

== matlab function simulation_model/Battery/Model/Aging Model/Aging factor Calculation Block/MATLAB Function1 ==
  data: N1 input; Nmax input; Epsi output; Nmaxprev input; DOD1 input; DOD2 input; DOD3 input; c input; Epsiprev input; EpsiEqprev input; EpsiEq output; Ageprev input; Age output
function [Epsi,EpsiEq,Age] = fcn(N1,Nmax, Nmaxprev,DOD1,DOD2,DOD3,c,Epsiprev,EpsiEqprev,Ageprev)
%#codegen
 Epsi = Epsiprev;
 EpsiEq = EpsiEqprev;
 Age = Ageprev;
if(c>=3)
if (Nmax==Nmaxprev)
    Epsi = Epsiprev;
    EpsiEq = EpsiEqprev;
    Age = Ageprev;
else 
    Epsi = Epsiprev+(0.5/Nmax)*(1-(DOD3/DOD2))+(0.5/Nmax)*(1-(DOD1/DOD2));
    Age = Epsi*N1;
end
end

== matlab function simulation_model/Charging//Discharging Controller/MATLAB Function ==
  data: ibatt output; Idis input; Icharge input; Stateprev input; State output; SoC input; cycleprev input; cycle output
function [ibatt,State,cycle] = fcn(Idis,Icharge,Stateprev,SoC,cycleprev)
%#codegen
State=Stateprev;
cycle=cycleprev;

if(Stateprev==1 && SoC==0)
    State=0;
    cycle=cycleprev+1;
end

if(Stateprev==0 && SoC==100)
    State=1;
end

if (Stateprev==1)
  ibatt=Idis;
else
  ibatt=-Icharge;
end

== matlab function simulation_model/Battery/Model/Aging Model/DOD and average current calculation Block ==
  data: dSOC_dT output; ibatdAv output; ibatcAv output; ibat input; SOC input; ndprev input; ncprev input; ibattTdprev input; ibattTcprev input; ibatcAv1prev input; ibatdAv1prev input; ibatdAv2prev input; IdAveprev input; IcAveprev input; nd output; nc output; ibattTd output; ibattTc output; ibatcAv1 output; ibatdAv1 output; ibatdAv2 output; IdAve output; IcAve output; SOCdprev input; SOCd output; DODd output; DODdn1 output; DODdn2 output; DOD1 output; DOD2 output; DOD3 output; c output; DODdprev input; DODdn1prev input; DODdn2prev input; DOD1prev input; DOD2prev input; DOD3prev input; cprev input; Stateprev input; State output
function [dSOC_dT,ibatdAv,ibatcAv,nd,nc,ibattTd,ibattTc,ibatcAv1,ibatdAv1,ibatdAv2,IdAve,IcAve,SOCd,DODd,DODdn1,DODdn2,DOD1,DOD2,DOD3,c,State] = fcn(ibat,SOC,ndprev,ncprev,ibattTdprev,ibattTcprev,ibatcAv1prev,ibatdAv1prev,ibatdAv2prev,IdAveprev,IcAveprev,SOCdprev, DODdprev,DODdn1prev,DODdn2prev,DOD1prev, DOD2prev,DOD3prev,cprev,Stateprev)
%#codegen
DOD = 100 - SOC;
dSOC_dT= (SOC-SOCdprev);
SOCd = SOC;
nd=ndprev+1;
nc=ncprev+1;
if(dSOC_dT <=0)
    s=0;
else
    s=1;
end
IdAve=IdAveprev;
IcAve=IcAveprev;
if(s==0)
ibattTd=ibattTdprev+abs(ibat);
ibatdAv =ibattTd/nd;
IdAve = ibatdAv;
ibattTc=0;
nc=0;
ibatcAv=0;
else
    ibattTd=0;
    nd=0;
    ibatdAv=0;
    ibattTc=ibattTcprev+abs(ibat);
    ibatcAv =ibattTc/nc;
    IcAve=ibatcAv;
end
sprev = Stateprev;
c=cprev;
if (s==sprev)
    DODdn2 = DODdn2prev;
    DODdn1 = DODdn1prev;
    DODd=DODdprev;
else
    DODd = DOD;
    c=cprev+1;
    DODdn2 = DODdn1prev;
    DODdn1 = DODdprev;
end
State=s;
ibatdAv2=ibatdAv2prev;
if(mod(c,2)==0)
    ibatdAv2=IdAveprev;
end
DOD1=DOD1prev;
DOD2=DOD2prev;
DOD3=DOD3prev;
ibatcAv1=ibatcAv1prev;
ibatdAv1=ibatdAv1prev;
if(mod(c,2)>0)
    DOD1=DODd;
    DOD2=DODdn1;
    DOD3=DODdn2;
    ibatcAv1=IcAve;
    ibatdAv1=ibatdAv2;
end
